simulink model "OL_model_control_synthesis_paper_SAuncertain_add_mul_noweights"  (R2020b)
settings: Solver=VariableStepAuto  StartTime=0.0  StopTime=10.0  RelTol=1e-3
libraries: cstblocks x4, RCTblocks x1
settings Model: Creator=T.FORMOSA  LastModifiedBy=ricardorodrigues
settings DebuggingCC: AlgebraicLoopMsg=none  ArithmeticOperatorsInVariantConditions=warning
settings SFSimCC: CustomCodeUndefinedFunction=UseInterfaceOnly

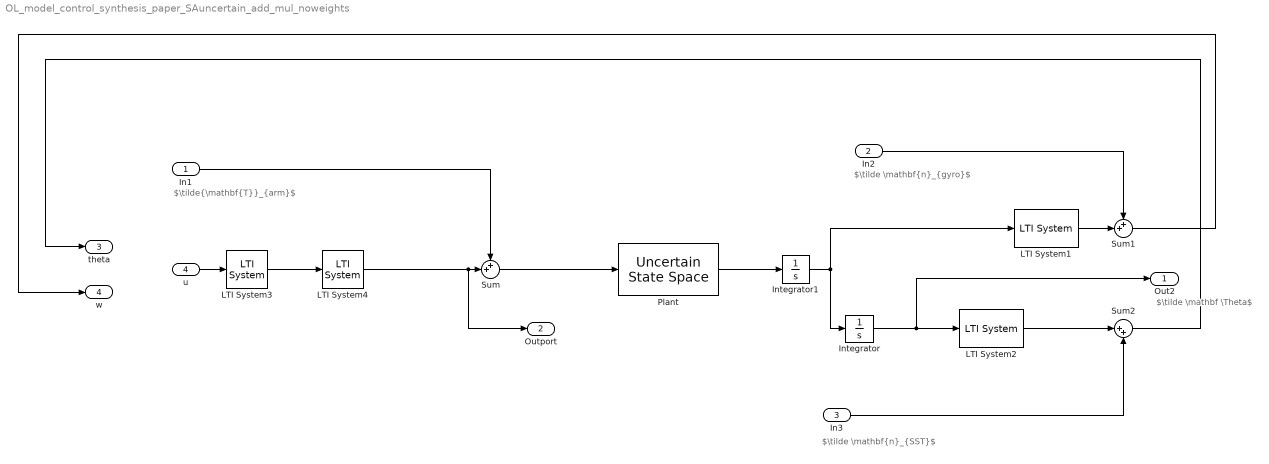
== system OL_model_control_synthesis_paper_SAuncertain_add_mul_noweights ==
  note: $\tilde \mathbf{n}_{SST}$
  note: $\tilde \mathbf{n}_{gyro}$
  note: $\tilde \mathbf \Theta$
  note: $\tilde{\mathbf{T}}_{arm}$
  In1 : Inport  PortDimensions=3
  In2 : Inport  Port=2  PortDimensions=3
  In3 : Inport  Port=3  PortDimensions=3
  u : Inport  Port=4
  Integrator : Integrator
  Integrator1 : Integrator
  LTI System1 : cstblocks/LTI System  sys=GYRO  IC=[]
  LTI System2 : cstblocks/LTI System  sys=SST  IC=[]
  LTI System3 : cstblocks/LTI System  sys=rolloff  IC=[]
  LTI System4 : cstblocks/LTI System  sys=RW  IC=[]
  Plant : RCTblocks/Uncertain State Space  Tag=USS  SCDEnableBlockLinearizationSpecification=on  USystem=PlantU  UValue=[]  X0=[]  uX0=[]
      settings: SourceProductBaseCode=RC
  Sum : Sum  Inputs=++|
  Sum1 : Sum  Inputs=++|
  Sum2 : Sum  Inputs=|++
  Out2 : Outport  VectorParamsAs1DForOutWhenUnconnected=off
  Outport : Outport  Port=2
  theta : Outport  Port=3
  w : Outport  Port=4
  wires:
  Integrator1/1 -> LTI System1/1, Integrator/1
  LTI System1/1 -> Sum1/2
  Sum2/1 -> theta/1
  LTI System2/1 -> Sum2/1
  Integrator/1 -> Out2/1, LTI System2/1
  Sum1/1 -> w/1
  Sum/1 -> Plant/1
  Plant/1 -> Integrator1/1
  u/1 -> LTI System3/1
  In1/1 -> Sum/1
  In2/1 -> Sum1/1
  In3/1 -> Sum2/2
  LTI System3/1 -> LTI System4/1
  LTI System4/1 -> Outport/1, Sum/2
